simulink model "FSAC2021_V1"  (R2014a)
settings: Solver=FixedStepDiscrete  StartTime=0.0  StopTime=inf  FixedStep=0.0005  RelTol=1e-3
model workspace (MAT data in the model file):
  MCOS : class17 (value not decoded)
  MCOS : class17 (value not decoded)
  MCOS : class17 (value not decoded)
  MCOS : class17 (value not decoded)
  MCOS : class17 (value not decoded)
  MCOS : class17 (value not decoded)
  MCOS : class17 (value not decoded)
  MCOS : class17 (value not decoded)
  MCOS : class17 (value not decoded)
  MCOS : class17 (value not decoded)
  MCOS : class17 (value not decoded)
  MCOS : class17 (value not decoded)
  MCOS : class17 (value not decoded)
  MCOS : class17 (value not decoded)
  MCOS : class17 (value not decoded)
  MCOS : class17 (value not decoded)
  MCOS : class17 (value not decoded)
  MCOS : class17 (value not decoded)
  MCOS : class17 (value not decoded)
  BUZZER_START = 1
  MCOS : class17 (value not decoded)
  MCOS : class17 (value not decoded)
  MCOS : class17 (value not decoded)
  MCOS : class17 (value not decoded)
  MCOS : class17 (value not decoded)
  MCOS : class17 (value not decoded)
  MCOS : class17 (value not decoded)
  MCOS : class17 (value not decoded)
  MCOS : class17 (value not decoded)
  MCOS : class17 (value not decoded)
  MCOS : class17 (value not decoded)
  MCOS : class17 (value not decoded)
  MCOS : class17 (value not decoded)
  MCOS : class17 (value not decoded)
  MCOS : class17 (value not decoded)
  MCOS : class17 (value not decoded)
  MCOS : class17 (value not decoded)
  MCOS : class17 (value not decoded)
  MCOS : class17 (value not decoded)
  MCOS : class17 (value not decoded)
  MCOS : class17 (value not decoded)
  MCOS : class17 (value not decoded)
  MCOS : class17 (value not decoded)
  MCOS : class17 (value not decoded)
  MCOS : class17 (value not decoded)
  MCOS : class17 (value not decoded)
  MCOS : class17 (value not decoded)
  MCOS : class17 (value not decoded)
  MCOS : class17 (value not decoded)
  MCOS : class17 (value not decoded)
  MCOS : class17 (value not decoded)
  MCOS : class17 (value not decoded)
  MCOS : class17 (value not decoded)
  MCOS : class17 (value not decoded)
  MCOS : class17 (value not decoded)
  MCOS : class17 (value not decoded)
  MCOS : class17 (value not decoded)
  MCOS : class17 (value not decoded)
  Brake = 11
  MCOS : class17 (value not decoded)
  MCOS : class17 (value not decoded)
  MCOS : class17 (value not decoded)
  MCOS : class17 (value not decoded)
  MCOS : class17 (value not decoded)
  MCOS : class17 (value not decoded)
  MCOS : class17 (value not decoded)
  MCOS : class17 (value not decoded)
  Sensor_Acc_b = 101.85
  Sensor_Acc_k = -0.0185
  Str_Sen_Orig_Angle = -341
  MCOS : class17 (value not decoded)
  Tire_D = 0.47
  T = 0.05
libraries: simulink x189, ec55xxlib x135
(part 2 of 9)

== system FSAC2021_V1/CAN_SEND/Subsystem2 ==
  Brk_Mtr_GoalPos : Inport
  Acc_Cmd : Inport  Port=2
  function : TriggerPort  TriggerType=function-call
  BCU_MTR_MOVE_AB : Subsystem
  CANTransmit3 : ec55xxlib/RapidECU_U2/07CANCommucation/CANTransmit  canmodule=A  canbuffer=58  canmessageid=358  canmessagetype=Standard(11-bit ID)  datalength=4  sampletime=-1
  CANTransmit4 : ec55xxlib/RapidECU_U2/07CANCommucation/CANTransmit  canmodule=B  canbuffer=15  canmessageid=2197885092  canmessagetype=Extended(29-bit ID)  datalength=2  sampletime=-1
  Data Type Conversion17 : DataTypeConversion
  MOTOR_SPEED_CONTROL : Subsystem
  MeaModule : ec55xxlib/RapidECU_U2/11Calibration/MeaModule  signal=To_MOTOR_OK
  MeaModule1 : ec55xxlib/RapidECU_U2/11Calibration/MeaModule  signal=ACC
  MeaModule8 : ec55xxlib/RapidECU_U2/11Calibration/MeaModule  signal=pulses
  Terminator3 : Terminator
  Terminator4 : Terminator
  wires:
  Brk_Mtr_GoalPos/1 -> MeaModule8/1
  MOTOR_SPEED_CONTROL/1(output) -> CANTransmit4/1
  MeaModule1/1 -> MOTOR_SPEED_CONTROL/1(Drive_Speed_Control_in)
  MeaModule/1 -> Terminator4/1
  Acc_Cmd/1 -> MeaModule1/1
  CANTransmit3/1 -> Terminator3/1
  BCU_MTR_MOVE_AB/1(output) -> CANTransmit3/1
  CANTransmit4/1 -> MeaModule/1
  Data Type Conversion17/1 -> BCU_MTR_MOVE_AB/1(Brake_mtr_goalpos_in)
  MeaModule8/1 -> Data Type Conversion17/1

== system FSAC2021_V1/CAN_SEND/Subsystem3 ==
  BCU_STATUS_READ : Subsystem
  CANTransmit1 : ec55xxlib/RapidECU_U2/07CANCommucation/CANTransmit  canmodule=B  canbuffer=13  canmessageid=2181107875  canmessagetype=Extended(29-bit ID)  datalength=8  sampletime=0.05
  CANTransmit6 : ec55xxlib/RapidECU_U2/07CANCommucation/CANTransmit  canmodule=A  canbuffer=59  canmessageid=382  canmessagetype=Standard(11-bit ID)  datalength=2  sampletime=0.01
  Constant : Constant  Value=2
  Constant1 : Constant
  Data Type Conversion : DataTypeConversion
  MOTOR_READ_SPEED : Subsystem
  MeaModule1 : ec55xxlib/RapidECU_U2/11Calibration/MeaModule  signal=read_speed
  MeaModule2 : ec55xxlib/RapidECU_U2/11Calibration/MeaModule  signal=Read_BCU
  Terminator1 : Terminator
  Terminator6 : Terminator
  wires:
  CANTransmit6/1 -> MeaModule2/1
  Constant/1 -> BCU_STATUS_READ/1(status_reg_num_in)
  Constant1/1 -> BCU_STATUS_READ/2(status_reg_addr_start_in)
  BCU_STATUS_READ/1(output) -> CANTransmit6/1
  MeaModule2/1 -> Terminator6/1
  MOTOR_READ_SPEED/1(output) -> Data Type Conversion/1
  CANTransmit1/1 -> MeaModule1/1
  Data Type Conversion/1 -> CANTransmit1/1
  MeaModule1/1 -> Terminator1/1

== system FSAC2021_V1/Controller/200ms_Duty ==
  LED_Blue_Flag : Inport
  LED_Yellow_Flag : Inport  Port=2
  Buzzer_Flag : Inport  Port=3
  function : TriggerPort  TriggerType=function-call
  Light_Subsystem : Subsystem  TreatAsAtomicUnit=on
  Light_Subsystem1 : Subsystem  TreatAsAtomicUnit=on
  Light_Subsystem2 : Subsystem  TreatAsAtomicUnit=on
  MeaModule : ec55xxlib/RapidECU_U2/11Calibration/MeaModule  signal=blue
  Blue_Light_Pin : Outport
  Yellow_Light_Pin : Outport  Port=2
  Buzzer_Pin : Outport  Port=3
  Buzzer_Overflag : Outport  Port=4
  wires:
  LED_Yellow_Flag/1 -> Light_Subsystem1/1(Light_Status)
  Light_Subsystem1/1(Light_Output) -> Yellow_Light_Pin/1
  LED_Blue_Flag/1 -> Light_Subsystem/1(Light_Status)
  Light_Subsystem/1(Light_Output) -> MeaModule/1
  Buzzer_Flag/1 -> Light_Subsystem2/1(Buzzer_Flag)
  Light_Subsystem2/1(Buzzer_Pin) -> Buzzer_Pin/1
  Light_Subsystem2/2(Buzzer_Overflag) -> Buzzer_Overflag/1
  MeaModule/1 -> Blue_Light_Pin/1

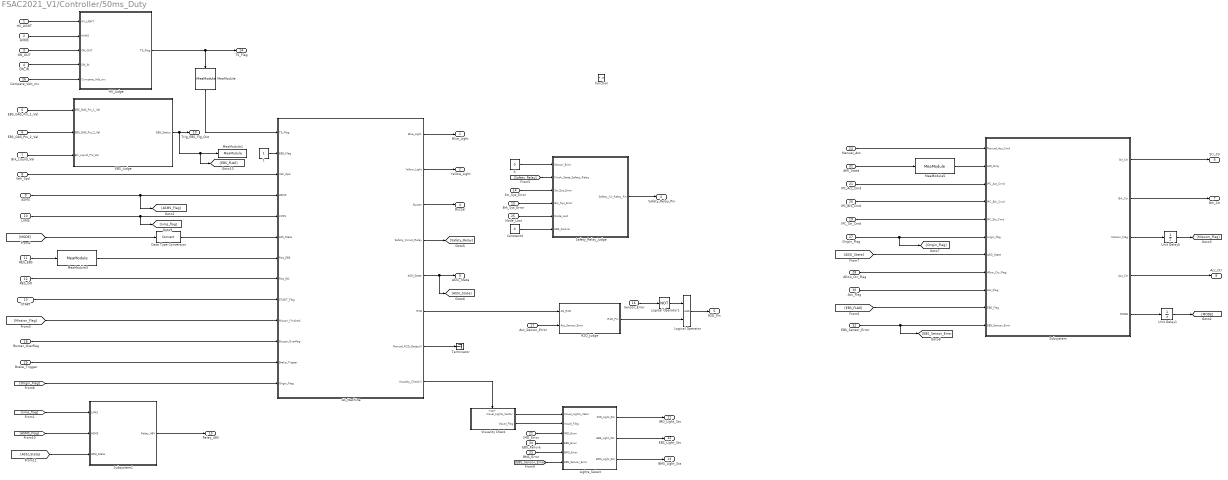
== system FSAC2021_V1/Controller/50ms_Duty ==
  HV_LIGHT : Inport
  HVMS : Inport  Port=2
  ON_OUT : Inport  Port=3
  ON_IN : Inport  Port=4
  EBS_GAS_Prs_1_Val : Inport  Port=5
  EBS_GAS_Prs_2_Val : Inport  Port=6
  Brk_Liquid_Val : Inport  Port=7
  Veh_Spd : Inport  Port=8
  ASMS : Inport  Port=9
  LVMS : Inport  Port=10
  RES_EBS : Inport  Port=11
  RES_GO : Inport  Port=12
  START : Inport  Port=13
  Str_Sys_Error : Inport  Port=14
  Brk_Sys_Error : Inport  Port=15
  Sensor_Error : Inport  Port=16
  Acc_Sensor_Error : Inport  Port=17
  Buzzer_Overflag : Inport  Port=18
  IPC_Str_Cmd : Inport  Port=19
  IPC_Brk_Cmd : Inport  Port=20
  IPC_Acc_Cmd : Inport  Port=21
  IMD_Error : Inport  Port=22
  BMS_Error : Inport  Port=23
  Manual_Acc : Inport  Port=24
  Node_Lost : Inport  Port=25
  Compare_Volt_mv : Inport  Port=26
  Origin_Flag : Inport  Port=27
  Allow_Ctr_Flag : Inport  Port=28
  "Brake_Trigger " : Inport  Port=29
  Acc_Flag : Inport  Port=30
  AMI_State : Inport  Port=31
  EBS_Sensor_Error : Inport  Port=32
  EBS_Failure : Inport  Port=33
  function : TriggerPort  TriggerType=function-call
  1 : Constant  OutDataTypeStr=uint8
  4 : Constant  Value=0  OutDataTypeStr=uint8
  AS_Machine : Stateflow chart  TreatAsAtomicUnit=on
  Constant2 : Constant  Value=0
  Data Type Conversion : DataTypeConversion
  EBS_Judge : Subsystem
  "HV_Judge " : Subsystem
  Lights_Select : Subsystem
  Logical Operator : Logic  AllPortsSameDT=off  OutDataTypeStr=boolean
  Logical Operator1 : Logic  Operator=NOT  AllPortsSameDT=off  OutDataTypeStr=boolean
  MeaModule : ec55xxlib/RapidECU_U2/11Calibration/MeaModule  signal=TS_Flag
  MeaModule1 : ec55xxlib/RapidECU_U2/11Calibration/MeaModule  signal=EBS_Status
  MeaModule3 : ec55xxlib/RapidECU_U2/11Calibration/MeaModule  signal=RES_EBS
  MeaModule5 : ec55xxlib/RapidECU_U2/11Calibration/MeaModule  signal=AMI_State
  R2D_Judge : Subsystem
  Safety_Relay_Judge : Subsystem
  Subsystem : Subsystem
  Subsystem1 : Subsystem
  Terminator : Terminator
  Unit Delay1 : UnitDelay  SampleTime=-1
  Unit Delay5 : UnitDelay  SampleTime=-1
  Visuality Check : Subsystem  TreatAsAtomicUnit=on
  Blue_Light : Outport
  Yellow_Light : Outport  Port=2
  Buzzer : Outport  Port=3
  Safety_Relay_Pin : Outport  Port=4
  R2D_Pin : Outport  Port=5
  Str_Ctr : Outport  Port=6
  Brk_Ctr : Outport  Port=7
  Acc_Ctr : Outport  Port=8
  ASSI_State : Outport  Port=9
  Trig_EBS_Flg_Out : Outport  Port=10
  IMD_Light_Sts : Outport  Port=11
  EBS_Light_Sts : Outport  Port=12
  BMS_Light_Sts : Outport  Port=13
  TS_Flag : Outport  Port=14
  Relay_48V : Outport  Port=15
  wires:
  HV_LIGHT/1 -> "HV_Judge "/1(HV_LIGHT)
  HVMS/1 -> "HV_Judge "/2(HVMS)
  EBS_GAS_Prs_2_Val/1 -> EBS_Judge/2(EBS_GAS_Prs_2_Val)
  EBS_GAS_Prs_1_Val/1 -> EBS_Judge/1(EBS_GAS_Prs_1_Val)
  EBS_Judge/1(EBS_Status) -> Trig_EBS_Flg_Out/1, [EBS_FLAG], MeaModule1/1
  ASMS/1 -> [ASMS_Flag], AS_Machine/4(ASMS)
  LVMS/1 -> [lvms_flag], AS_Machine/5(LVMS)
  ON_OUT/1 -> "HV_Judge "/3(ON_OUT)
  AS_Machine/2(Yellow_Light) -> Yellow_Light/1
  AS_Machine/1(Blue_Light) -> Blue_Light/1
  AS_Machine/3(Buzzer) -> Buzzer/1
  AS_Machine/6(R2D) -> R2D_Judge/1(AS_R2D)
  Buzzer_Overflag/1 -> AS_Machine/11(Buzzer_Overflag)
  ON_IN/1 -> "HV_Judge "/4(ON_IN)
  RES_EBS/1 -> MeaModule3/1
  Safety_Relay_Judge/1(Safety_Cir_Relay_Pin) -> Safety_Relay_Pin/1
  Acc_Sensor_Error/1 -> R2D_Judge/2(Acc_Sensor_Error)
  IPC_Str_Cmd/1 -> Subsystem/5(IPC_Str_Cmd)
  IPC_Brk_Cmd/1 -> Subsystem/4(IPC_Brk_Cmd)
  IPC_Acc_Cmd/1 -> Subsystem/3(IPC_Acc_Cmd)
  Subsystem/1(Str_Ctr) -> Str_Ctr/1
  Subsystem/2(Brk_Ctr) -> Brk_Ctr/1
  Brk_Liquid_Val/1 -> EBS_Judge/3(Brk_Liquid_Prs_Val)
  Visuality Check/1(Visual_Lights_Vector) -> Lights_Select/1(Visual_Lights_Vetor)
  Visuality Check/2(Visual_Flag) -> Lights_Select/2(Visual_Flag)
  IMD_Error/1 -> Lights_Select/3(IMD_Error)
  EBS_Failure/1 -> Lights_Select/4(EBS_Error)
  BMS_Error/1 -> Lights_Select/5(BMS_Error)
  Lights_Select/2(EBS_Light_Sts) -> EBS_Light_Sts/1
  Lights_Select/1(IMD_Light_Sts) -> IMD_Light_Sts/1
  Lights_Select/3(BMS_Light_Sts) -> BMS_Light_Sts/1
  AS_Machine/8(Visuality_Check()) -> Visuality Check/Trigger
  Manual_Acc/1 -> Subsystem/1(Manual_Acc_Cmd)
  AS_Machine/5(ASSI_State) -> [ASSI_State], ASSI_State/1
  Str_Sys_Error/1 -> Safety_Relay_Judge/3(Str_Sys_Error)
  Brk_Sys_Error/1 -> Safety_Relay_Judge/4(Brk_Sys_Error)
  Veh_Spd/1 -> AS_Machine/3(Veh_Spd)
  MeaModule/1 -> AS_Machine/1(TS_Flag)
  Compare_Volt_mv/1 -> "HV_Judge "/5(Compare_Volt_mv)
  "HV_Judge "/1(TS_Flag) -> MeaModule/1, TS_Flag/1
  START/1 -> AS_Machine/9(START_Flag)
  Origin_Flag/1 -> [Origin_Flag], Subsystem/6(origin_flag)
  Unit Delay5/1 -> [Mission_Flag]
  Subsystem/4(Acc_Ctr) -> Acc_Ctr/1
  RES_GO/1 -> AS_Machine/8(Res_GO)
  MeaModule3/1 -> AS_Machine/7(Res_EBS)
  [Mission_Flag] -> AS_Machine/10(Misson_Finished)
  Subsystem/3(Mission_Flag) -> Unit Delay5/1
  "Brake_Trigger "/1 -> AS_Machine/12(Brake_Trigeer)
  Constant2/1 -> Safety_Relay_Judge/6(EBS_Failure)
  Acc_Flag/1 -> Subsystem/9(Acc_Flag)
  R2D_Judge/1(R2D_Pin) -> Logical Operator/2
  Logical Operator/1 -> R2D_Pin/1
  Sensor_Error/1 -> Logical Operator1/1
  Logical Operator1/1 -> Logical Operator/1
  Allow_Ctr_Flag/1 -> Subsystem/8(Allow_Ctr_Flag)
  4/1 -> Safety_Relay_Judge/1(Sensor_Error)
  AS_Machine/4(Safety_Circuit_Relay) -> [Safety_Relay]
  [Safety_Relay] -> Safety_Relay_Judge/2(Finish_State_Safety_Relay)
  [ASSI_State] -> Subsystem/7(ASSI_State)
  AMI_State/1 -> MeaModule5/1
  MeaModule5/1 -> Subsystem/2(AMI_Duty)
  Subsystem/5(MODE) -> Unit Delay1/1
  Unit Delay1/1 -> [MODE]
  [MODE] -> Data Type Conversion/1
  Data Type Conversion/1 -> AS_Machine/6(AMI_State)
  [Origin_Flag] -> AS_Machine/13(Origin_Flag)
  EBS_Sensor_Error/1 -> [EBS_Sensor_Error], Subsystem/11(EBS_Sensor_Error)
  [EBS_Sensor_Error] -> Lights_Select/6(EBS_Sensor_Error)
  Node_Lost/1 -> Safety_Relay_Judge/5(Node_Lost)
  [lvms_flag] -> Subsystem1/1(LVMS)
  [ASMS_Flag] -> Subsystem1/2(ASMS)
  [ASSI_State] -> Subsystem1/3(ASSI_State)
  Subsystem1/1(Relay_48V) -> Relay_48V/1
  [EBS_FLAG] -> Subsystem/10(EBS_Flag)
  AS_Machine/7(Manual_R2D_Detect()) -> Terminator/1
  1/1 -> AS_Machine/2(EBS_Flag)

== system FSAC2021_V1/Controller/BCU_Controller ==
  note: 任何控制源禁止在Allow_Ctrl_Flg未置1的时候控制车辆
  Brk_Cmd : Inport
  Brk_Mtr_Enable_Flg : Inport  Port=2
  ASSI_State : Inport  Port=3
  function : TriggerPort  TriggerType=function-call
  BCU_Strategy : Stateflow chart
  Brk_Move : Subsystem
  Constant1 : Constant
  MeaModule : ec55xxlib/RapidECU_U2/11Calibration/MeaModule  signal=Brk_Enable_Flag
  Allow_Ctrl_Flg : Outport
  Brk_Mtr_Origin_funCall : Outport  Port=2
  Brk_Mtr_Enable_funCall : Outport  Port=3
  Brk_Mtr_GoalPos : Outport  Port=4
  wires:
  Brk_Mtr_Enable_Flg/1 -> MeaModule/1
  Constant1/1 -> BCU_Strategy/3(Brk_Mtr_Origin_Flag)
  BCU_Strategy/2(Brk_Ctrl_State) -> Brk_Move/1(Brk_Ctrl_State)
  ASSI_State/1 -> BCU_Strategy/2(ASSI_State)
  BCU_Strategy/1(Allow_Ctrl_Flg) -> Allow_Ctrl_Flg/1
  BCU_Strategy/3(Brk_Mtr_BackOrigin()) -> Brk_Mtr_Origin_funCall/1
  BCU_Strategy/4(Brk_Mtr_Enable()) -> Brk_Mtr_Enable_funCall/1
  Brk_Move/1(Brk_Mtr_GoalPos) -> Brk_Mtr_GoalPos/1
  Brk_Cmd/1 -> Brk_Move/2(Brk_Cmd)
  MeaModule/1 -> BCU_Strategy/1(Brk_Mtr_Enable_Flg)

== system FSAC2021_V1/Controller/SteerCtr ==
  Str_Snr_Ang : Inport
  Steer_Cmd : Inport  Port=2
  Str_Status : Inport  Port=3
  ASSI_State : Inport  Port=4
  function : TriggerPort  TriggerType=function-call
  Chart : Stateflow chart  SystemSampleTime=0.01
  Data Type Conversion{,1..3} (4 alike) : DataTypeConversion
  MeaModule : ec55xxlib/RapidECU_U2/11Calibration/MeaModule  signal=Back_Angle
  MeaModule1 : ec55xxlib/RapidECU_U2/11Calibration/MeaModule  signal=enflag
  MeaModule2 : ec55xxlib/RapidECU_U2/11Calibration/MeaModule  signal=flag
  MeaModule3 : ec55xxlib/RapidECU_U2/11Calibration/MeaModule  signal=Str
  Subsystem3 : Subsystem
  Terminator : Terminator
  Terminator1 : Terminator
  NMT_nodeorder : Outport
  NMT_nodectrl : Outport  Port=2
  Enable_Operation_Ctrl : Outport  Port=3
  Quick_Stop_Ctrl : Outport  Port=4
  Enable_Voltage_Ctrl : Outport  Port=5
  Halt_Ctrl : Outport  Port=6
  Switch_On_Ctrl : Outport  Port=7
  Abs_or_Rel_Ctrl : Outport  Port=8
  New_Set_Point_Ctrl : Outport  Port=9
  Position_set : Outport  Port=10
  Encoder_Msg_Data : Outport  Port=11
  TmtNNMTCAN : Outport  Port=12
  TmtRPDO1CAN : Outport  Port=13
  TmtSDOCAN : Outport  Port=14
  Original_Flag : Outport  Port=15
  Fault_Reset : Outport  Port=16
  wires:
  Str_Status/1 -> Data Type Conversion1/1
  Data Type Conversion3/1 -> Subsystem3/1(In1)
  ASSI_State/1 -> Data Type Conversion/1
  Data Type Conversion2/1 -> MeaModule3/1
  Data Type Conversion/1 -> Chart/3(ASSI_State)
  Data Type Conversion1/1 -> Chart/4(Str_Status)
  Chart/1(NMT_nodeorder) -> NMT_nodeorder/1
  Chart/2(NMT_nodectrl) -> NMT_nodectrl/1
  Chart/3(Enable_Operation_Ctrl) -> Enable_Operation_Ctrl/1
  Chart/4(Quick_Stop_Ctrl) -> Quick_Stop_Ctrl/1
  Chart/5(Enable_Voltage_Ctrl) -> Enable_Voltage_Ctrl/1
  Chart/6(Halt_Ctrl) -> Halt_Ctrl/1
  Chart/7(Switch_On_Ctrl) -> Switch_On_Ctrl/1
  Chart/8(Abs_or_Rel_Ctrl) -> Abs_or_Rel_Ctrl/1
  Chart/9(New_Set_Point_Ctrl) -> New_Set_Point_Ctrl/1
  Chart/11(Encoder_Msg_Data) -> Encoder_Msg_Data/1
  Chart/12(Original_Flag) -> Original_Flag/1
  Chart/16(TmtNMTCAN()) -> TmtNNMTCAN/1
  Chart/17(TmtRPDO1CAN()) -> TmtRPDO1CAN/1
  Chart/18(TmtSDOCAN()) -> TmtSDOCAN/1
  Subsystem3/1(Out1) -> MeaModule/1
  MeaModule/1 -> Chart/1(Origin_Back_Angle)
  Str_Snr_Ang/1 -> Data Type Conversion3/1
  Chart/13(Fault_Resrt) -> Fault_Reset/1
  Chart/10(Position_set) -> Position_set/1
  Chart/14(flag) -> MeaModule2/1
  MeaModule2/1 -> Terminator/1
  MeaModule3/1 -> Chart/2(Steer_Go_Angle)
  Chart/15(enflag) -> MeaModule1/1
  MeaModule1/1 -> Terminator1/1
  Steer_Cmd/1 -> Data Type Conversion2/1

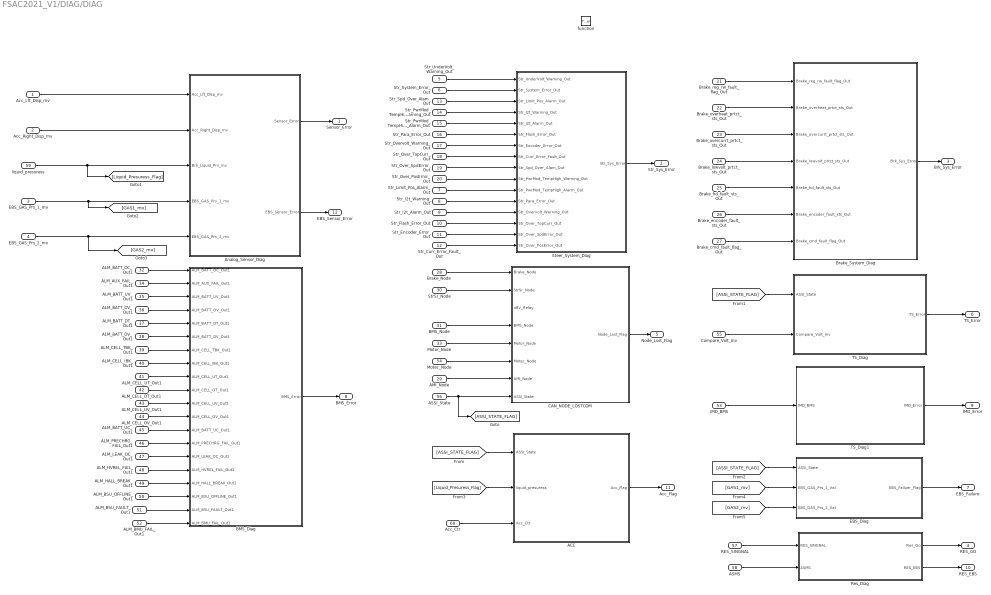
== system FSAC2021_V1/DIAG/DIAG ==
  Acc_Lft_Disp_mv : Inport
  Acc_Right_Disp_mv : Inport  Port=2
  EBS_GAS_Prs_1_mv : Inport  Port=3
  EBS_GAS_Prs_2_mv : Inport  Port=4
  Str_UnderVolt_Warning_Out : Inport  Port=5
  Str_System_Error_Out : Inport  Port=6
  Str_Limit_Pos_Alarm_Out : Inport  Port=7
  Str_I2t_Warning_Out : Inport  Port=8
  Str_I2t_Alarm_Out : Inport  Port=9
  Str_Flash_Error_Out : Inport  Port=10
  Str_Encoder_Error_Out : Inport  Port=11
  Str_Curr_Error_Fault_Out : Inport  Port=12
  Str_Spd_Over_Alam_Out : Inport  Port=13
  Str_PwrMod_TempHigh_Warning_Out : Inport  Port=14
  Str_PwrMod_TempHigh_Alarm_Out : Inport  Port=15
  Str_Para_Error_Out : Inport  Port=16
  Str_Overvolt_Warning_Out : Inport  Port=17
  Str_Over_TopCurr_Out : Inport  Port=18
  Str_Over_SpdError_Out : Inport  Port=19
  Str_Over_PosError_Out : Inport  Port=20
  Brake_reg_rw_fault_flag_Out : Inport  Port=21
  Brake_overheat_prtct_sts_Out : Inport  Port=22
  Brake_overcurrt_prtct_sts_Out : Inport  Port=23
  Brake_lowvolt_prtct_sts_Out : Inport  Port=24
  Brake_hd_fault_sts_Out : Inport  Port=25
  Brake_encoder_fault_sts_Out : Inport  Port=26
  Brake_cmd_fault_flag_Out : Inport  Port=27
  Brake_Node : Inport  Port=28
  AMI_Node : Inport  Port=29
  StrSr_Node : Inport  Port=30
  BMS_Node : Inport  Port=31
  ALM_BATT_OC_Out1 : Inport  Port=32
  Motor_Node : Inport  Port=33
  ALM_AUX_FAIL_Out1 : Inport  Port=34
  ALM_BATT_UV_Out1 : Inport  Port=35
  ALM_BATT_OV_Out1 : Inport  Port=36
  ALM_BATT_DT_Out1 : Inport  Port=37
  ALM_BATT_DV_Out1 : Inport  Port=38
  ALM_CELL_TBK_Out1 : Inport  Port=39
  ALM_CELL_IBK_Out1 : Inport  Port=40
  ALM_CELL_UT_Out1 : Inport  Port=41
  ALM_CELL_OT_Out1 : Inport  Port=42
  ALM_CELL_UV_Out1 : Inport  Port=43
  ALM_CELL_OV_Out1 : Inport  Port=44
  ALM_BATT_UC_Out1 : Inport  Port=45
  ALM_PRECHRG_FAIL_Out1 : Inport  Port=46
  ALM_LEAK_OC_Out1 : Inport  Port=47
  ALM_HVREL_FAIL_Out1 : Inport  Port=48
  ALM_HALL_BREAK_Out1 : Inport  Port=49
  ALM_BSU_OFFLINE_Out1 : Inport  Port=50
  ALM_BSU_FAULT_Out1 : Inport  Port=51
  ALM_BMU_FAIL_Out1 : Inport  Port=52
  "IMD_BMS " : Inport  Port=53
  Motec_Node : Inport  Port=54
  Compare_Volt_mv : Inport  Port=55
  ASSI_State : Inport  Port=56
  RES_SINGNAL : Inport  Port=57
  ASMS : Inport  Port=58
  liquid_presuress : Inport  Port=59
  Acc_Ctr : Inport  Port=60
  function : TriggerPort  TriggerType=function-call
  ACC : Subsystem
  Analog_Sensor_Diag : Subsystem
  BMS_Diag : Subsystem
  Brake_System_Diag : Subsystem
  CAN_NODE_LOSTCOM : Subsystem
  EBS_Diag : Subsystem
  Res_Diag : Subsystem
  Steer_System_Diag : Subsystem
  TS_Diag : Subsystem
  TS_Diag1 : Subsystem
  Sensor_Error : Outport
  Str_Sys_Error : Outport  Port=2
  Brk_Sys_Error : Outport  Port=3
  RES_GO : Outport  Port=4
  Node_Lost_Flag : Outport  Port=5
  TS_Error : Outport  Port=6
  EBS_Failure : Outport  Port=7
  "BMS_Error " : Outport  Port=8
  IMD_Error : Outport  Port=9
  RES_EBS : Outport  Port=10
  Acc_Flag : Outport  Port=11
  EBS_Sensor_Error : Outport  Port=12
  wires:
  Str_UnderVolt_Warning_Out/1 -> Steer_System_Diag/1(Str_UnderVolt_Warning_Out)
  Str_System_Error_Out/1 -> Steer_System_Diag/2(Str_System_Error_Out)
  Str_Spd_Over_Alam_Out/1 -> Steer_System_Diag/3(Str_Limit_Pos_Alarm_Out)
  Str_PwrMod_TempHigh_Warning_Out/1 -> Steer_System_Diag/4(Str_I2t_Warning_Out)
  Str_PwrMod_TempHigh_Alarm_Out/1 -> Steer_System_Diag/5(Str_I2t_Alarm_Out)
  Str_Overvolt_Warning_Out/1 -> Steer_System_Diag/7(Str_Encoder_Error_Out)
  Str_Over_TopCurr_Out/1 -> Steer_System_Diag/8(Str_Curr_Error_Fault_Out)
  Str_Para_Error_Out/1 -> Steer_System_Diag/6(Str_Flash_Error_Out)
  Str_Over_SpdError_Out/1 -> Steer_System_Diag/9(Str_Spd_Over_Alam_Out)
  Str_Over_PosError_Out/1 -> Steer_System_Diag/10(Str_PwrMod_TempHigh_Warning_Out)
  Str_Limit_Pos_Alarm_Out/1 -> Steer_System_Diag/11(Str_PwrMod_TempHigh_Alarm_Out)
  Str_I2t_Warning_Out/1 -> Steer_System_Diag/12(Str_Para_Error_Out)
  Str_I2t_Alarm_Out/1 -> Steer_System_Diag/13(Str_Overvolt_Warning_Out)
  Str_Flash_Error_Out/1 -> Steer_System_Diag/14(Str_Over_TopCurr_Out)
  Str_Encoder_Error_Out/1 -> Steer_System_Diag/15(Str_Over_SpdError_Out)
  Str_Curr_Error_Fault_Out/1 -> Steer_System_Diag/16(Str_Over_PosError_Out)
  Steer_System_Diag/1(Str_Sys_Error) -> Str_Sys_Error/1
  Brake_overcurrt_prtct_sts_Out/1 -> Brake_System_Diag/3(Brake_overcurrt_prtct_sts_Out)
  Brake_overheat_prtct_sts_Out/1 -> Brake_System_Diag/2(Brake_overheat_prtct_sts_Out)
  Brake_lowvolt_prtct_sts_Out/1 -> Brake_System_Diag/4(Brake_lowvolt_prtct_sts_Out)
  Brake_reg_rw_fault_flag_Out/1 -> Brake_System_Diag/1(Brake_reg_rw_fault_flag_Out)
  Brake_hd_fault_sts_Out/1 -> Brake_System_Diag/5(Brake_hd_fault_sts_Out)
  Brake_encoder_fault_sts_Out/1 -> Brake_System_Diag/6(Brake_encoder_fault_sts_Out)
  Brake_cmd_fault_flag_Out/1 -> Brake_System_Diag/7(Brake_cmd_fault_flag_Out)
  Brake_System_Diag/1(Brk_Sys_Error) -> Brk_Sys_Error/1
  Acc_Right_Disp_mv/1 -> Analog_Sensor_Diag/2(Acc_Right_Disp_mv)
  Acc_Lft_Disp_mv/1 -> Analog_Sensor_Diag/1(Acc_Lft_Disp_mv)
  Analog_Sensor_Diag/1(Sensor_Error) -> Sensor_Error/1
  CAN_NODE_LOSTCOM/1(Node_Lost_Flag) -> Node_Lost_Flag/1
  TS_Diag/1(TS_Error) -> TS_Error/1
  EBS_GAS_Prs_1_mv/1 -> Analog_Sensor_Diag/4(EBS_GAS_Prs_1_mv), [GAS1_mv]
  EBS_GAS_Prs_2_mv/1 -> [GAS2_mv], Analog_Sensor_Diag/5(EBS_GAS_Prs_2_mv)
  EBS_Diag/1(EBS_Failuer_Flag) -> EBS_Failure/1
  ASSI_State/1 -> [ASSI_STATE_FLAG], CAN_NODE_LOSTCOM/8(ASSI_State)
  ALM_BATT_OC_Out1/1 -> BMS_Diag/1(ALM_BATT_OC_Out1)
  ALM_AUX_FAIL_Out1/1 -> BMS_Diag/2(ALM_AUX_FAIL_Out1)
  ALM_BATT_UV_Out1/1 -> BMS_Diag/3(ALM_BATT_UV_Out1)
  ALM_BATT_OV_Out1/1 -> BMS_Diag/4(ALM_BATT_OV_Out1)
  ALM_BATT_DT_Out1/1 -> BMS_Diag/5(ALM_BATT_DT_Out1)
  ALM_BATT_DV_Out1/1 -> BMS_Diag/6(ALM_BATT_DV_Out1)
  ALM_CELL_TBK_Out1/1 -> BMS_Diag/7(ALM_CELL_TBK_Out1)
  ALM_CELL_IBK_Out1/1 -> BMS_Diag/8(ALM_CELL_IBK_Out1)
  ALM_CELL_UT_Out1/1 -> BMS_Diag/9(ALM_CELL_UT_Out1)
  ALM_CELL_OT_Out1/1 -> BMS_Diag/10(ALM_CELL_OT_Out1)
  ALM_CELL_UV_Out1/1 -> BMS_Diag/11(ALM_CELL_UV_Out1)
  ALM_CELL_OV_Out1/1 -> BMS_Diag/12(ALM_CELL_OV_Out1)
  ALM_BATT_UC_Out1/1 -> BMS_Diag/13(ALM_BATT_UC_Out1)
  ALM_PRECHRG_FAIL_Out1/1 -> BMS_Diag/14(ALM_PRECHRG_FAIL_Out1)
  ALM_LEAK_OC_Out1/1 -> BMS_Diag/15(ALM_LEAK_OC_Out1)
  ALM_HVREL_FAIL_Out1/1 -> BMS_Diag/16(ALM_HVREL_FAIL_Out1)
  ALM_HALL_BREAK_Out1/1 -> BMS_Diag/17(ALM_HALL_BREAK_Out1)
  ALM_BSU_OFFLINE_Out1/1 -> BMS_Diag/18(ALM_BSU_OFFLINE_Out1)
  ALM_BSU_FAULT_Out1/1 -> BMS_Diag/19(ALM_BSU_FAULT_Out1)
  ALM_BMU_FAIL_Out1/1 -> BMS_Diag/20(ALM_BMU_FAIL_Out1)
  BMS_Diag/1("BMS_Error ") -> "BMS_Error "/1
  "IMD_BMS "/1 -> TS_Diag1/1("IMD_BMS ")
  TS_Diag1/1(IMD_Error) -> IMD_Error/1
  Brake_Node/1 -> CAN_NODE_LOSTCOM/1(Brake_Node)
  Motor_Node/1 -> CAN_NODE_LOSTCOM/5(Motor_Node)
  StrSr_Node/1 -> CAN_NODE_LOSTCOM/2(StrSr_Node)
  BMS_Node/1 -> CAN_NODE_LOSTCOM/4(BMS_Node)
  Motec_Node/1 -> CAN_NODE_LOSTCOM/6(Motec_Node)
  Compare_Volt_mv/1 -> TS_Diag/2(Compare_Volt_mv)
  AMI_Node/1 -> CAN_NODE_LOSTCOM/7(AMI_Node)
  Res_Diag/1(Res_Go) -> RES_GO/1
  RES_SINGNAL/1 -> Res_Diag/1(RES_SINGNAL)
  ASMS/1 -> Res_Diag/2(ASMS)
  Res_Diag/2(RES_EBS) -> RES_EBS/1
  Acc_Ctr/1 -> ACC/3(Acc_Ctr)
  ACC/1(Acc_Flag) -> Acc_Flag/1
  liquid_presuress/1 -> Analog_Sensor_Diag/3(Brk_Liquid_Prs_mv), [Liquid_Presuress_Flag]
  Analog_Sensor_Diag/2(EBS_Sensor_Error) -> EBS_Sensor_Error/1
  [ASSI_STATE_FLAG] -> ACC/1(ASSI_State)
  [ASSI_STATE_FLAG] -> TS_Diag/1(ASSI_State)
  [ASSI_STATE_FLAG] -> EBS_Diag/1(ASSI_State)
  [Liquid_Presuress_Flag] -> ACC/2(liquid_presuress)
  [GAS1_mv] -> EBS_Diag/2(EBS_GAS_Prs_1_Val)
  [GAS2_mv] -> EBS_Diag/3(EBS_GAS_Prs_2_Val)

== system FSAC2021_V1/I//O_OutPut/Subsystem ==
  Blue_Light_Pin : Inport
  Yellow_Light_Pin : Inport  Port=2
  Buzzer_pin : Inport  Port=3
  Safety_Relay_Pin : Inport  Port=4
  Relay_48V_Pin : Inport  Port=5
  R2D_pin : Inport  Port=6
  IMD_Light : Inport  Port=7
  EBS_Light : Inport  Port=8
  BMS_Light : Inport  Port=9
  Liquid_Pressure : Inport  Port=10
  function : TriggerPort  TriggerType=function-call
  48V_Relay : ec55xxlib/RapidECU_U2/04PowerDriverSwitch/PowerDriverSwitch  channel=59: O_PWM2_LS1A8  sampletime=-1
  Blue_Pin : ec55xxlib/RapidECU_U2/04PowerDriverSwitch/PowerDriverSwitch  channel=114: O_PWM9_HS2A9  sampletime=-1
  Buzzer_Pin : ec55xxlib/RapidECU_U2/04PowerDriverSwitch/PowerDriverSwitch  channel=117: O_PWM11_HS2A9  sampletime=-1
  Compare To Constant : simulink/Logic and Bit Operations/Compare To Constant  relop=>=  const=30  OutDataTypeStr=boolean
  Constant : Constant
  Constant1 : Constant  Value=0
  Data Type Conversion{,1..4,6..10} (10 alike) : DataTypeConversion  OutDataTypeStr=boolean
  MeaModule : ec55xxlib/RapidECU_U2/11Calibration/MeaModule  signal=Stafe_Relay_pin
  MeaModule1 : ec55xxlib/RapidECU_U2/11Calibration/MeaModule  signal=R2D_Voltage
  MeaModule2 : ec55xxlib/RapidECU_U2/11Calibration/MeaModule  signal=Buzzer_pin
  MeaModule3 : ec55xxlib/RapidECU_U2/11Calibration/MeaModule  signal=V48_relay
  MeaModule4 : ec55xxlib/RapidECU_U2/11Calibration/MeaModule  signal=IMD
  MeaModule5 : ec55xxlib/RapidECU_U2/11Calibration/MeaModule  signal=EBS
  MeaModule6 : ec55xxlib/RapidECU_U2/11Calibration/MeaModule  signal=BMS_LIGHT
  MeaModule7 : ec55xxlib/RapidECU_U2/11Calibration/MeaModule  signal=light_blue
  MeaModule8 : ec55xxlib/RapidECU_U2/11Calibration/MeaModule  signal=brake_light
  R2D_Pin : ec55xxlib/RapidECU_U2/04PowerDriverSwitch/PowerDriverSwitch  channel=61: O_PWM4_LS1A8  sampletime=-1
  "Safety_Relay " : ec55xxlib/RapidECU_U2/04PowerDriverSwitch/PowerDriverSwitch  channel=58: O_PWM1_LS1A8  sampletime=-1
  Switch : Switch  Criteria=u2 > Threshold
  VCU_Valve1 : ec55xxlib/RapidECU_U2/04PowerDriverSwitch/PowerDriverSwitch  channel=82: O_PWM5_LS1A8  sampletime=-1
  VCU_Valve2 : ec55xxlib/RapidECU_U2/04PowerDriverSwitch/PowerDriverSwitch  channel=90: O_PWM6_LS1A8  sampletime=-1
  VCU_Valve3 : ec55xxlib/RapidECU_U2/04PowerDriverSwitch/PowerDriverSwitch  channel=92: O_PWM7_LS1A8  sampletime=-1
  VCU_Valve4 : ec55xxlib/RapidECU_U2/04PowerDriverSwitch/PowerDriverSwitch  channel=118: O_PWM12_HS2A9  sampletime=-1
  Yellow_Pin : ec55xxlib/RapidECU_U2/04PowerDriverSwitch/PowerDriverSwitch  channel=115: O_PWM10_HS2A9  sampletime=-1
  wires:
  Data Type Conversion1/1 -> Yellow_Pin/1
  Blue_Light_Pin/1 -> Data Type Conversion/1
  Buzzer_pin/1 -> Data Type Conversion2/1
  Data Type Conversion2/1 -> MeaModule2/1
  Data Type Conversion3/1 -> MeaModule/1
  Data Type Conversion4/1 -> MeaModule3/1
  Yellow_Light_Pin/1 -> Data Type Conversion1/1
  R2D_pin/1 -> Data Type Conversion6/1
  Data Type Conversion/1 -> MeaModule7/1
  Data Type Conversion9/1 -> MeaModule5/1
  MeaModule2/1 -> Buzzer_Pin/1
  EBS_Light/1 -> Data Type Conversion9/1
  BMS_Light/1 -> Data Type Conversion10/1
  Safety_Relay_Pin/1 -> Data Type Conversion3/1
  MeaModule/1 -> "Safety_Relay "/1
  Data Type Conversion8/1 -> MeaModule4/1
  MeaModule4/1 -> VCU_Valve1/1
  MeaModule3/1 -> 48V_Relay/1
  MeaModule5/1 -> VCU_Valve2/1
  MeaModule6/1 -> VCU_Valve3/1
  IMD_Light/1 -> Data Type Conversion8/1
  Data Type Conversion6/1 -> MeaModule1/1
  Data Type Conversion10/1 -> MeaModule6/1
  MeaModule1/1 -> R2D_Pin/1
  Relay_48V_Pin/1 -> Data Type Conversion4/1
  MeaModule7/1 -> Blue_Pin/1
  Data Type Conversion7/1 -> MeaModule8/1
  Switch/1 -> Data Type Conversion7/1
  Liquid_Pressure/1 -> Compare To Constant/1
  Compare To Constant/1 -> Switch/2
  Constant/1 -> Switch/1
  Constant1/1 -> Switch/3
  MeaModule8/1 -> VCU_Valve4/1

== system FSAC2021_V1/Input_Process/KL_Sig_Process ==
  FL_WhlSpd_Hz : Inport
  FR_WhlSpd_Hz : Inport  Port=2
  RL_WhlSpd_Hz : Inport  Port=3
  RR_WhlSpd_Hz : Inport  Port=4
  Acc_Lft_Disp_mv : Inport  Port=5
  Acc_Right_Disp_mv : Inport  Port=6
  Brk_Liquid_Prs_mv : Inport  Port=7
  EBS_GAS_Prs_1_mv : Inport  Port=8
  EBS_GAS_Prs_2_mv : Inport  Port=9
  function : TriggerPort  TriggerType=function-call
  Analog_Signal_Process : Subsystem
  Whl_Spd_Process : Subsystem
  Vel_Spd : Outport
  Whl_Spd_FL_Val : Outport  Port=2
  Whl_Spd_FF_Val : Outport  Port=3
  Whl_Spd_RL_Val : Outport  Port=4
  Whl_Spd_RR_Val : Outport  Port=5
  Acc_Lft_Disp_Val : Outport  Port=6
  Acc_Right_Disp_Val : Outport  Port=7
  Brk_Liquid_Prs_Val : Outport  Port=8
  EBS_GAS_Prs_1_Val : Outport  Port=9
  EBS_GAS_Prs_2_Val : Outport  Port=10
  ACC : Outport  Port=11
  wires:
  Whl_Spd_Process/2(Whl_Spd_FL_Val) -> Whl_Spd_FL_Val/1
  Whl_Spd_Process/3(Whl_Spd_FF_Val) -> Whl_Spd_FF_Val/1
  Whl_Spd_Process/4(Whl_Spd_RL_Val) -> Whl_Spd_RL_Val/1
  Whl_Spd_Process/5(Whl_Spd_RR_Val) -> Whl_Spd_RR_Val/1
  Whl_Spd_Process/1(Vel_Spd) -> Vel_Spd/1
  RR_WhlSpd_Hz/1 -> Whl_Spd_Process/4(RR_WhlSpd_Hz)
  RL_WhlSpd_Hz/1 -> Whl_Spd_Process/3(RL_WhlSpd_Hz)
  FR_WhlSpd_Hz/1 -> Whl_Spd_Process/2(FR_WhlSpd_Hz)
  FL_WhlSpd_Hz/1 -> Whl_Spd_Process/1(FL_WhlSpd_Hz)
  Analog_Signal_Process/3(Brk_Liquid_Prs_Val) -> Brk_Liquid_Prs_Val/1
  Analog_Signal_Process/4(EBS_GAS_Prs_1_Val) -> EBS_GAS_Prs_1_Val/1
  Analog_Signal_Process/5(EBS_GAS_Prs_2_Val) -> EBS_GAS_Prs_2_Val/1
  EBS_GAS_Prs_2_mv/1 -> Analog_Signal_Process/5(EBS_GAS_Prs_2_mv)
  EBS_GAS_Prs_1_mv/1 -> Analog_Signal_Process/4(EBS_GAS_Prs_1_mv)
  Brk_Liquid_Prs_mv/1 -> Analog_Signal_Process/3(Brk_Liquid_Prs_mv)
  Acc_Lft_Disp_mv/1 -> Analog_Signal_Process/1(Acc_Lft_Disp_mv)
  Acc_Right_Disp_mv/1 -> Analog_Signal_Process/2(Acc_Right_Disp_mv)
  Analog_Signal_Process/2(Acc_Right_Disp_Val) -> Acc_Right_Disp_Val/1
  Analog_Signal_Process/1(Acc_Lft_Disp_Val) -> Acc_Lft_Disp_Val/1
  Analog_Signal_Process/6(ACC) -> ACC/1

== system FSAC2021_V1/VCU_CAN_Read/PCANA(RES、AMI、MOTEC、BRAKE、STEER_SENSOR、IPC) ==
  function : TriggerPort  TriggerType=function-call
  BCU_MTR_STATUS : ec55xxlib/RapidECU_U2/07CANCommucation/CANReceive  canmodule=A  canbuffer=21  canmessageid=257  canmessagetype=Standard(11-bit ID)  datalength=8  sampletime=-1
  BCU_MTR_STATUS1 : Subsystem
  Data Type Conversion{1..21} (21 alike) : DataTypeConversion
  IPC_CMD1 : Subsystem
  MOTEC_MOTION1 : ec55xxlib/RapidECU_U2/07CANCommucation/CANReceive  canmodule=A  canbuffer=41  canmessageid=256  canmessagetype=Standard(11-bit ID)  datalength=3  sampletime=-1
  MOTEC_MOTION2 : ec55xxlib/RapidECU_U2/07CANCommucation/CANReceive  canmodule=A  canbuffer=35  canmessageid=279  canmessagetype=Standard(11-bit ID)  datalength=1  sampletime=-1
  MeaModule2 : ec55xxlib/RapidECU_U2/11Calibration/MeaModule  signal=brake_node
  MeaModule3 : ec55xxlib/RapidECU_U2/11Calibration/MeaModule  signal=strsr_node
  MeaModule4 : ec55xxlib/RapidECU_U2/11Calibration/MeaModule  signal=RES_Value
  MeaModule5 : ec55xxlib/RapidECU_U2/11Calibration/MeaModule  signal=RES__ok
  MeaModule6 : ec55xxlib/RapidECU_U2/11Calibration/MeaModule  signal=Steer_sensor_angle
  Res_Message1 : Subsystem
  STEER_SENSOR_INFO1 : Subsystem
  Steer_Sensor : ec55xxlib/RapidECU_U2/07CANCommucation/CANReceive  canmodule=A  canbuffer=38  canmessageid=485  canmessagetype=Standard(11-bit ID)  datalength=8  sampletime=-1
  Subsystem : Subsystem
  Terminator{1,3,11,13..20} (11 alike) : Terminator
  StrSr_Node : Outport
  StrSr_Snr_Ang : Outport  Port=2
  Brake_mtr_goalpos_Out : Outport  Port=3
  Brake_speed_enqual_Out : Outport  Port=4
  Brake_pos_enqual_Out : Outport  Port=5
  Brake_sensor6_sts_Out : Outport  Port=6
  Brake_sensor5_sts_Out : Outport  Port=7
  Brake_sensor4_sts_Out : Outport  Port=8
  Brake_sensor3_sts_Out : Outport  Port=9
  Brake_sensor2_sts_Out : Outport  Port=10
  Brake_sensor1_sts_Out : Outport  Port=11
  Brake_reg_rw_fault_flag_Out : Outport  Port=12
  Brake_overheat_prtct_sts_Out : Outport  Port=13
  Brake_overcurrt_prtct_sts_Out : Outport  Port=14
  Brake_offline_run_flag_O : Outport  Port=15
  Brake_mtr_stop_flag_Out : Outport  Port=16
  Brake_mtr_origin_flag_Out : Outport  Port=17
  Brake_mtr_enable_flag_Out : Outport  Port=18
  Brake_lowvolt_prtct_sts_Out : Outport  Port=19
  Brake_hd_fault_sts_Out : Outport  Port=20
  Brake_go_origin_over_flag_Out : Outport  Port=21
  Brake_encoder_fault_sts_Out : Outport  Port=22
  Brake_cmd_fault_flag_Out : Outport  Port=23
  Brk_Node : Outport  Port=24
  IPC_Steer : Outport  Port=25
  IPC_Brk : Outport  Port=26
  IPC_Acc : Outport  Port=27
  RES_Signal : Outport  Port=28
  wires:
  Steer_Sensor/1 -> STEER_SENSOR_INFO1/Trigger
  Steer_Sensor/4 -> STEER_SENSOR_INFO1/1(input)
  Steer_Sensor/2 -> MeaModule3/1
  STEER_SENSOR_INFO1/1(Str_Sensor_Curr_Angle_Out) -> MeaModule6/1
  Steer_Sensor/3 -> Terminator11/1
  Steer_Sensor/5 -> Terminator15/1
  MeaModule3/1 -> StrSr_Node/1
  MeaModule6/1 -> StrSr_Snr_Ang/1
  BCU_MTR_STATUS1/13(Brake_offline_run_flag_Out) -> Data Type Conversion13/1
  BCU_MTR_STATUS1/2(Brake_speed_enqual_Out) -> Data Type Conversion2/1
  BCU_MTR_STATUS/5 -> Terminator20/1
  BCU_MTR_STATUS1/16(Brake_mtr_enable_flag_Out) -> Data Type Conversion16/1
  BCU_MTR_STATUS/3 -> Terminator19/1
  BCU_MTR_STATUS/2 -> MeaModule2/1
  BCU_MTR_STATUS1/5(Brake_sensor5_sts_Out) -> Data Type Conversion5/1
  BCU_MTR_STATUS1/14(Brake_mtr_stop_flag_Out) -> Data Type Conversion14/1
  BCU_MTR_STATUS1/17(Brake_lowvolt_prtct_sts_Out) -> Data Type Conversion17/1
  BCU_MTR_STATUS/4 -> BCU_MTR_STATUS1/1(input)
  BCU_MTR_STATUS1/1(Brake_mtr_goalpos_Out) -> Data Type Conversion1/1
  BCU_MTR_STATUS1/18(Brake_hd_fault_sts_Out) -> Data Type Conversion18/1
  BCU_MTR_STATUS1/12(Brake_overcurrt_prtct_sts_Out) -> Data Type Conversion12/1
  BCU_MTR_STATUS1/19(Brake_go_origin_over_flag_Out) -> Data Type Conversion19/1
  BCU_MTR_STATUS/1 -> BCU_MTR_STATUS1/Trigger
  BCU_MTR_STATUS1/6(Brake_sensor4_sts_Out) -> Data Type Conversion6/1
  BCU_MTR_STATUS1/4(Brake_sensor6_sts_Out) -> Data Type Conversion4/1
  BCU_MTR_STATUS1/8(Brake_sensor2_sts_Out) -> Data Type Conversion8/1
  BCU_MTR_STATUS1/3(Brake_pos_enqual_Out) -> Data Type Conversion3/1
  BCU_MTR_STATUS1/10(Brake_reg_rw_fault_flag_Out) -> Data Type Conversion10/1
  BCU_MTR_STATUS1/20(Brake_encoder_fault_sts_Out) -> Data Type Conversion20/1
  BCU_MTR_STATUS1/21(Brake_cmd_fault_flag_Out) -> Data Type Conversion21/1
  BCU_MTR_STATUS1/9(Brake_sensor1_sts_Out) -> Data Type Conversion9/1
  BCU_MTR_STATUS1/15(Brake_mtr_origin_flag_Out) -> Data Type Conversion15/1
  BCU_MTR_STATUS1/11(Brake_overheat_prtct_sts_Out) -> Data Type Conversion11/1
  BCU_MTR_STATUS1/7(Brake_sensor3_sts_Out) -> Data Type Conversion7/1
  Data Type Conversion17/1 -> Brake_lowvolt_prtct_sts_Out/1
  Data Type Conversion1/1 -> Brake_mtr_goalpos_Out/1
  Data Type Conversion11/1 -> Brake_overheat_prtct_sts_Out/1
  Data Type Conversion13/1 -> Brake_offline_run_flag_O/1
  Data Type Conversion12/1 -> Brake_overcurrt_prtct_sts_Out/1
  Data Type Conversion10/1 -> Brake_reg_rw_fault_flag_Out/1
  Data Type Conversion16/1 -> Brake_mtr_enable_flag_Out/1
  Data Type Conversion14/1 -> Brake_mtr_stop_flag_Out/1
  Data Type Conversion18/1 -> Brake_hd_fault_sts_Out/1
  Data Type Conversion4/1 -> Brake_sensor6_sts_Out/1
  Data Type Conversion5/1 -> Brake_sensor5_sts_Out/1
  Data Type Conversion6/1 -> Brake_sensor4_sts_Out/1
  Data Type Conversion7/1 -> Brake_sensor3_sts_Out/1
  Data Type Conversion15/1 -> Brake_mtr_origin_flag_Out/1
  Data Type Conversion2/1 -> Brake_speed_enqual_Out/1
  Data Type Conversion8/1 -> Brake_sensor2_sts_Out/1
  Data Type Conversion19/1 -> Brake_go_origin_over_flag_Out/1
  Data Type Conversion9/1 -> Brake_sensor1_sts_Out/1
  Data Type Conversion21/1 -> Brake_cmd_fault_flag_Out/1
  Data Type Conversion3/1 -> Brake_pos_enqual_Out/1
  Data Type Conversion20/1 -> Brake_encoder_fault_sts_Out/1
  MeaModule2/1 -> Brk_Node/1
  MOTEC_MOTION1/4 -> IPC_CMD1/1(input)
  MOTEC_MOTION1/1 -> IPC_CMD1/Trigger
  MOTEC_MOTION1/3 -> Terminator3/1
  MOTEC_MOTION1/5 -> Terminator13/1
  Subsystem/3(Out3) -> IPC_Acc/1
  Subsystem/2(Out2) -> IPC_Brk/1
  IPC_CMD1/1(IPC_Steer_Out) -> Subsystem/1(In1)
  IPC_CMD1/2(IPC_Brk_Out) -> Subsystem/2(In2)
  IPC_CMD1/3(IPC_Acc_Out) -> Subsystem/3(In3)
  MOTEC_MOTION1/2 -> Subsystem/Enable
  Subsystem/1(Out1) -> IPC_Steer/1
  MOTEC_MOTION2/1 -> Res_Message1/Trigger
  MOTEC_MOTION2/2 -> MeaModule5/1
  MOTEC_MOTION2/3 -> Terminator14/1
  MOTEC_MOTION2/4 -> Res_Message1/1(input)
  MOTEC_MOTION2/5 -> Terminator16/1
  Res_Message1/1(Safety_Relay_Out) -> Terminator17/1
  Res_Message1/3(Res_check_Out) -> Terminator18/1
  Res_Message1/2(Res_Run_Status_Out) -> MeaModule4/1
  MeaModule4/1 -> RES_Signal/1
  MeaModule5/1 -> Terminator1/1

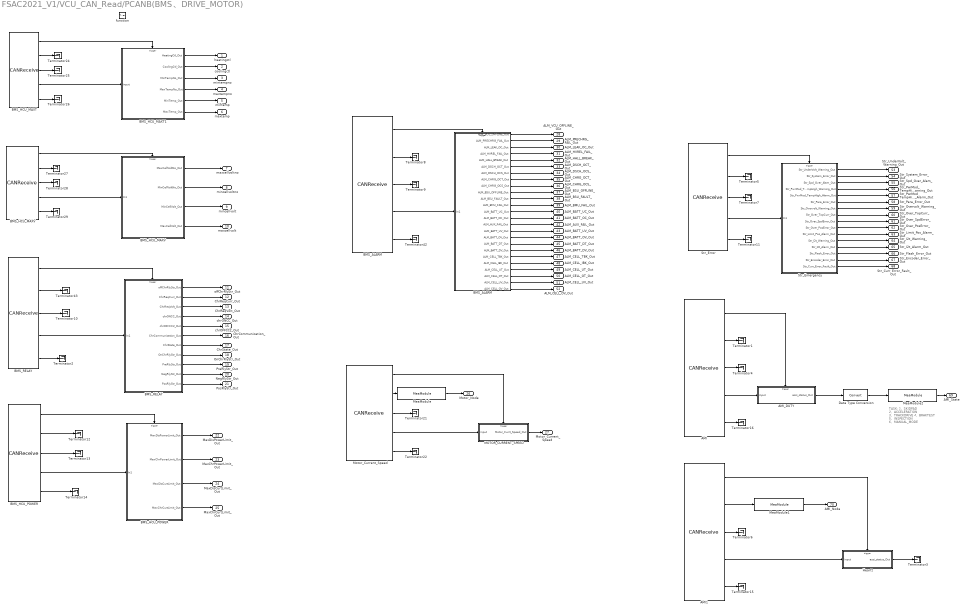
== system FSAC2021_V1/VCU_CAN_Read/PCANB(BMS、DRIVE_MOTOR) ==
  note: TASK:
      | 1、SKIDPAD
      | 2、ACCELERATION
      | 3、TRACKDRIVE
      | 4、BRAKTEST
      | 5、INSPECTION
      | 6、MANUAL_MODE
  function : TriggerPort  TriggerType=function-call
  AMI : ec55xxlib/RapidECU_U2/07CANCommucation/CANReceive  canmodule=A  canbuffer=16  canmessageid=1169  canmessagetype=Standard(11-bit ID)  datalength=1  sampletime=-1
  AMI1 : ec55xxlib/RapidECU_U2/07CANCommucation/CANReceive  canmodule=A  canbuffer=26  canmessageid=1168  canmessagetype=Standard(11-bit ID)  datalength=1  sampletime=-1
  AMI_DUTY : Subsystem
  BMS_ALARM : ec55xxlib/RapidECU_U2/07CANCommucation/CANReceive  canmodule=B  canbuffer=50  canmessageid=2556772595  canmessagetype=Extended(29-bit ID)  datalength=8  sampletime=-1
  "BMS_ALARM " : Subsystem
  BMS_HCU_MAXT : ec55xxlib/RapidECU_U2/07CANCommucation/CANReceive  canmodule=B  canbuffer=18  canmessageid=2556575987  canmessagetype=Extended(29-bit ID)  datalength=8  sampletime=-1
  BMS_HCU_MAXT1 : Subsystem
  BMS_HCU_MAXV : ec55xxlib/RapidECU_U2/07CANCommucation/CANReceive  canmodule=B  canbuffer=16  canmessageid=2556510451  canmessagetype=Extended(29-bit ID)  datalength=8  sampletime=-1
  "BMS_HCU_MAXV " : Subsystem
  BMS_HCU_POWER : ec55xxlib/RapidECU_U2/07CANCommucation/CANReceive  canmodule=B  canbuffer=52  canmessageid=2556707059  canmessagetype=Extended(29-bit ID)  datalength=8  sampletime=-1
  "BMS_HCU_POWER " : Subsystem
  BMS_RELAY : ec55xxlib/RapidECU_U2/07CANCommucation/CANReceive  canmodule=B  canbuffer=51  canmessageid=2556641523  canmessagetype=Extended(29-bit ID)  datalength=8  sampletime=-1
  "BMS_RELAY " : Subsystem
  Data Type Conversion : DataTypeConversion
  Heartt : Subsystem
  MOTOR_CURRENT_SPEED : Subsystem
  MeaModule : ec55xxlib/RapidECU_U2/11Calibration/MeaModule  signal=motor_node
  MeaModule1 : ec55xxlib/RapidECU_U2/11Calibration/MeaModule  signal=AMI_HEART
  MeaModule2 : ec55xxlib/RapidECU_U2/11Calibration/MeaModule  signal=AMI
  "Motor_Current_Speed " : ec55xxlib/RapidECU_U2/07CANCommucation/CANReceive  canmodule=B  canbuffer=21  canmessageid=2147553443  canmessagetype=Extended(29-bit ID)  datalength=2  sampletime=-1
  "Str_Emergency " : Subsystem
  Str_Error : ec55xxlib/RapidECU_U2/07CANCommucation/CANReceive  canmodule=A  canbuffer=4  canmessageid=129  canmessagetype=Standard(11-bit ID)  datalength=8  sampletime=-1
  Terminator{1..16,21..22,24..29,42..43} (26 alike) : Terminator
  heatingctl : Outport
  coolingctl : Outport  Port=2
  mintempno : Outport  Port=3
  maxtempno : Outport  Port=4
  mintemp : Outport  Port=5
  maxtemp : Outport  Port=6
  maxcellvoltno : Outport  Port=7
  mincellvoltno : Outport  Port=8
  mincellvolt : Outport  Port=9
  maxcellvolt : Outport  Port=10
  offChrRlyStr_Out : Outport  Port=11
  ChrReqCurr_Out : Outport  Port=12
  ChrReqVolt_Out : Outport  Port=13
  chrONCC_Out : Outport  Port=14
  chrOFFCC2_Out : Outport  Port=15
  ChrCommunication_Out : Outport  Port=16
  ChrState_Out : Outport  Port=17
  OnChrRlyStr_Out : Outport  Port=18
  PreRlyStr_Out : Outport  Port=19
  NegRlyStr_Out : Outport  Port=20
  PosRlyStr_Out : Outport  Port=21
  MaxDisPowerLimit_Out : Outport  Port=22
  MaxChrPowerLimit_Out : Outport  Port=23
  MaxDisCurtLimit_Out : Outport  Port=24
  MaxChrCurtLimit_Out : Outport  Port=25
  Motor_Node : Outport  Port=26
  Motor_Current_Speed : Outport  Port=27
  ALM_VCU_OFFLINE_Out : Outport  Port=28
  ALM_PRECHRG_FAIL_Out : Outport  Port=29
  ALM_LEAK_OC_Out : Outport  Port=30
  ALM_HVREL_FAIL_Out : Outport  Port=31
  ALM_HALL_BREAK_Out : Outport  Port=32
  ALM_DSCH_OCT_Out : Outport  Port=33
  ALM_DSCH_OCS_Out : Outport  Port=34
  ALM_CHRG_OCT_Out : Outport  Port=35
  ALM_CHRG_OCS_Out : Outport  Port=36
  ALM_BSU_OFFLINE_Out : Outport  Port=37
  ALM_BSU_FAULT_Out : Outport  Port=38
  ALM_BMU_FAIL_Out : Outport  Port=39
  ALM_BATT_UC_Out : Outport  Port=40
  ALM_BATT_OC_Out : Outport  Port=41
  ALM_AUX_FAIL_Out : Outport  Port=42
  ALM_BATT_UV_Out : Outport  Port=43
  ALM_BATT_OV_Out : Outport  Port=44
  ALM_BATT_DT_Out : Outport  Port=45
  ALM_BATT_DV_Out : Outport  Port=46
  ALM_CELL_TBK_Out : Outport  Port=47
  ALM_CELL_IBK_Out : Outport  Port=48
  ALM_CELL_UT_Out : Outport  Port=49
  ALM_CELL_OT_Out : Outport  Port=50
  ALM_CELL_UV_Out : Outport  Port=51
  ALM_CELL_OV_Out : Outport  Port=52
  Str_UnderVolt_Warning_Out : Outport  Port=53
  Str_System_Error_Out : Outport  Port=54
  Str_Spd_Over_Alam_Out : Outport  Port=55
  Str_PwrMod_TempHigh_Warning_Out : Outport  Port=56
  Str_PwrMod_TempHigh_Alarm_Out : Outport  Port=57
  Str_Para_Error_Out : Outport  Port=58
  Str_Overvolt_Warning_Out : Outport  Port=59
  Str_Over_TopCurr_Out : Outport  Port=60
  Str_Over_SpdError_Out : Outport  Port=61
  Str_Over_PosError_Out : Outport  Port=62
  Str_Limit_Pos_Alarm_Out : Outport  Port=63
  Str_I2t_Warning_Out : Outport  Port=64
  Str_I2t_Alarm_Out : Outport  Port=65
  Str_Flash_Error_Out : Outport  Port=66
  Str_Encoder_Error_Out : Outport  Port=67
  Str_Curr_Error_Fault_Out : Outport  Port=68
  AMI_State : Outport  Port=69
  AMI_Node : Outport  Port=70
  wires:
  BMS_ALARM/5 -> Terminator42/1
  BMS_ALARM/1 -> "BMS_ALARM "/Trigger
  BMS_ALARM/3 -> Terminator9/1
  BMS_ALARM/2 -> Terminator8/1
  BMS_ALARM/4 -> "BMS_ALARM "/1(In1)
  BMS_RELAY/1 -> "BMS_RELAY "/Trigger
  BMS_RELAY/3 -> Terminator10/1
  BMS_RELAY/4 -> "BMS_RELAY "/1(In1)
  BMS_RELAY/5 -> Terminator2/1
  BMS_RELAY/2 -> Terminator43/1
  BMS_HCU_POWER/5 -> Terminator14/1
  BMS_HCU_POWER/2 -> Terminator12/1
  BMS_HCU_POWER/4 -> "BMS_HCU_POWER "/1(In1)
  BMS_HCU_POWER/3 -> Terminator13/1
  BMS_HCU_MAXT/3 -> Terminator25/1
  BMS_HCU_MAXT/2 -> Terminator24/1
  BMS_HCU_MAXT/5 -> Terminator26/1
  BMS_HCU_MAXT/1 -> BMS_HCU_MAXT1/Trigger
  BMS_HCU_MAXT/4 -> BMS_HCU_MAXT1/1(input)
  BMS_HCU_MAXV/4 -> "BMS_HCU_MAXV "/1(In1)
  BMS_HCU_MAXV/3 -> Terminator28/1
  BMS_HCU_MAXV/1 -> "BMS_HCU_MAXV "/Trigger
  BMS_HCU_MAXV/5 -> Terminator29/1
  BMS_HCU_MAXV/2 -> Terminator27/1
  BMS_HCU_POWER/1 -> "BMS_HCU_POWER "/Trigger
  "Motor_Current_Speed "/4 -> MOTOR_CURRENT_SPEED/1(input)
  "Motor_Current_Speed "/1 -> MOTOR_CURRENT_SPEED/Trigger
  "Motor_Current_Speed "/2 -> MeaModule/1
  "Motor_Current_Speed "/3 -> Terminator21/1
  "Motor_Current_Speed "/5 -> Terminator22/1
  BMS_HCU_MAXT1/1(HeatingCtl_Out) -> heatingctl/1
  BMS_HCU_MAXT1/2(CoolingCtl_Out) -> coolingctl/1
  BMS_HCU_MAXT1/3(MinTempNo_Out) -> mintempno/1
  BMS_HCU_MAXT1/4(MaxTempNo_Out) -> maxtempno/1
  BMS_HCU_MAXT1/5(MinTemp_Out) -> mintemp/1
  BMS_HCU_MAXT1/6(MaxTemp_Out) -> maxtemp/1
  "BMS_HCU_MAXV "/1(MaxCellVoltNo_Out) -> maxcellvoltno/1
  "BMS_HCU_MAXV "/3(MinCellVolt_Out) -> mincellvolt/1
  "BMS_HCU_MAXV "/4(MaxCellVolt_Out) -> maxcellvolt/1
  "BMS_HCU_MAXV "/2(MinCellVoltNo_Out) -> mincellvoltno/1
  "BMS_RELAY "/1(offChrRlyStr_Out) -> offChrRlyStr_Out/1
  "BMS_RELAY "/2(ChrReqCurr_Out) -> ChrReqCurr_Out/1
  "BMS_RELAY "/3(ChrReqVolt_Out) -> ChrReqVolt_Out/1
  "BMS_RELAY "/4(chrONCC_Out) -> chrONCC_Out/1
  "BMS_RELAY "/5(chrOFFCC2_Out) -> chrOFFCC2_Out/1
  "BMS_RELAY "/10(NegRlyStr_Out) -> NegRlyStr_Out/1
  "BMS_RELAY "/9(PreRlyStr_Out) -> PreRlyStr_Out/1
  "BMS_RELAY "/11(PosRlyStr_Out) -> PosRlyStr_Out/1
  "BMS_RELAY "/6(ChrCommunication_Out) -> ChrCommunication_Out/1
  "BMS_RELAY "/8(OnChrRlyStr_Out) -> OnChrRlyStr_Out/1
  "BMS_RELAY "/7(ChrState_Out) -> ChrState_Out/1
  "BMS_HCU_POWER "/3(MaxDisCurtLimit_Out) -> MaxDisCurtLimit_Out/1
  "BMS_HCU_POWER "/4(MaxChrCurtLimit_Out) -> MaxChrCurtLimit_Out/1
  "BMS_HCU_POWER "/1(MaxDisPowerLimit_Out) -> MaxDisPowerLimit_Out/1
  "BMS_HCU_POWER "/2(MaxChrPowerLimit_Out) -> MaxChrPowerLimit_Out/1
  MeaModule/1 -> Motor_Node/1
  MOTOR_CURRENT_SPEED/1(Motor_Currt_Speed_Out) -> Motor_Current_Speed/1
  "BMS_ALARM "/20(ALM_CELL_TBK_Out) -> ALM_CELL_TBK_Out/1
  "BMS_ALARM "/21(ALM_CELL_IBK_Out) -> ALM_CELL_IBK_Out/1
  "BMS_ALARM "/13(ALM_BATT_UC_Out) -> ALM_BATT_UC_Out/1
  "BMS_ALARM "/1(ALM_VCU_OFFLINE_Out) -> ALM_VCU_OFFLINE_Out/1
  "BMS_ALARM "/9(ALM_CHRG_OCS_Out) -> ALM_CHRG_OCS_Out/1
  "BMS_ALARM "/22(ALM_CELL_UT_Out) -> ALM_CELL_UT_Out/1
  "BMS_ALARM "/14(ALM_BATT_OC_Out) -> ALM_BATT_OC_Out/1
  "BMS_ALARM "/15(ALM_AUX_FAIL_Out) -> ALM_AUX_FAIL_Out/1
  "BMS_ALARM "/2(ALM_PRECHRG_FAIL_Out) -> ALM_PRECHRG_FAIL_Out/1
  "BMS_ALARM "/6(ALM_DSCH_OCT_Out) -> ALM_DSCH_OCT_Out/1
  "BMS_ALARM "/7(ALM_DSCH_OCS_Out) -> ALM_DSCH_OCS_Out/1
  "BMS_ALARM "/5(ALM_HALL_BREAK_Out) -> ALM_HALL_BREAK_Out/1
  "BMS_ALARM "/8(ALM_CHRG_OCT_Out) -> ALM_CHRG_OCT_Out/1
  "BMS_ALARM "/12(ALM_BMU_FAIL_Out) -> ALM_BMU_FAIL_Out/1
  "BMS_ALARM "/16(ALM_BATT_UV_Out) -> ALM_BATT_UV_Out/1
  "BMS_ALARM "/17(ALM_BATT_OV_Out) -> ALM_BATT_OV_Out/1
  "BMS_ALARM "/4(ALM_HVREL_FAIL_Out) -> ALM_HVREL_FAIL_Out/1
  "BMS_ALARM "/18(ALM_BATT_DT_Out) -> ALM_BATT_DT_Out/1
  "BMS_ALARM "/11(ALM_BSU_FAULT_Out) -> ALM_BSU_FAULT_Out/1
  "BMS_ALARM "/10(ALM_BSU_OFFLINE_Out) -> ALM_BSU_OFFLINE_Out/1
  "BMS_ALARM "/19(ALM_BATT_DV_Out) -> ALM_BATT_DV_Out/1
  "BMS_ALARM "/3(ALM_LEAK_OC_Out) -> ALM_LEAK_OC_Out/1
  "BMS_ALARM "/24(ALM_CELL_UV_Out) -> ALM_CELL_UV_Out/1
  "BMS_ALARM "/25(ALM_CELL_OV_Out) -> ALM_CELL_OV_Out/1
  "BMS_ALARM "/23(ALM_CELL_OT_Out) -> ALM_CELL_OT_Out/1
  AMI/2 -> Terminator1/1
  AMI/5 -> Terminator16/1
  AMI/1 -> AMI_DUTY/Trigger
  AMI_DUTY/1(assi_status_Out) -> Data Type Conversion/1
  Data Type Conversion/1 -> MeaModule2/1
  AMI/4 -> AMI_DUTY/1(input)
  AMI/3 -> Terminator4/1
  AMI1/4 -> Heartt/1(input)
  AMI1/3 -> Terminator6/1
  AMI1/5 -> Terminator15/1
  AMI1/1 -> Heartt/Trigger
  AMI1/2 -> MeaModule1/1
  Heartt/1(assi_status_Out) -> Terminator3/1
  "Str_Emergency "/3(Str_Spd_Over_Alam_Out) -> Str_Spd_Over_Alam_Out/1
  "Str_Emergency "/15(Str_Encoder_Error_Out) -> Str_Encoder_Error_Out/1
  "Str_Emergency "/2(Str_System_Error_Out) -> Str_System_Error_Out/1
  "Str_Emergency "/13(Str_I2t_Alarm_Out) -> Str_I2t_Alarm_Out/1
  "Str_Emergency "/6(Str_Para_Error_Out) -> Str_Para_Error_Out/1
  "Str_Emergency "/5(Str_PwrMod_TempHigh_Alarm_Out) -> Str_PwrMod_TempHigh_Alarm_Out/1
  "Str_Emergency "/12(Str_I2t_Warning_Out) -> Str_I2t_Warning_Out/1
  Str_Error/5 -> Terminator11/1
  "Str_Emergency "/10(Str_Over_PosError_Out) -> Str_Over_PosError_Out/1
  Str_Error/4 -> "Str_Emergency "/1(In1)
  Str_Error/2 -> Terminator5/1
  "Str_Emergency "/7(Str_Overvolt_Warning_Out) -> Str_Overvolt_Warning_Out/1
  "Str_Emergency "/1(Str_UnderVolt_Warning_Out) -> Str_UnderVolt_Warning_Out/1
  "Str_Emergency "/11(Str_Limit_Pos_Alarm_Out) -> Str_Limit_Pos_Alarm_Out/1
  "Str_Emergency "/9(Str_Over_SpdError_Out) -> Str_Over_SpdError_Out/1
  Str_Error/3 -> Terminator7/1
  "Str_Emergency "/4(Str_PwrMod_TempHigh_Warning_Out) -> Str_PwrMod_TempHigh_Warning_Out/1
  "Str_Emergency "/16(Str_Curr_Error_Fault_Out) -> Str_Curr_Error_Fault_Out/1
  "Str_Emergency "/8(Str_Over_TopCurr_Out) -> Str_Over_TopCurr_Out/1
  "Str_Emergency "/14(Str_Flash_Error_Out) -> Str_Flash_Error_Out/1
  Str_Error/1 -> "Str_Emergency "/Trigger
  MeaModule2/1 -> AMI_State/1
  MeaModule1/1 -> AMI_Node/1

== system FSAC2021_V1/VCU_CAN_Read/Subsystem ==
  function : TriggerPort  TriggerType=function-call
  BMS_HCU_INFO : ec55xxlib/RapidECU_U2/07CANCommucation/CANReceive  canmodule=B  canbuffer=54  canmessageid=2556444915  canmessagetype=Extended(29-bit ID)  datalength=8  sampletime=-1
  "BMS_HCU_INFO " : Subsystem
  MeaModule1 : ec55xxlib/RapidECU_U2/11Calibration/MeaModule  signal=bms_node
  Terminator16 : Terminator
  Terminator17 : Terminator
  BATLIFE : Outport
  BATALM : Outport  Port=2
  BATSTATE : Outport  Port=3
  BATSOH : Outport  Port=4
  BATSOC : Outport  Port=5
  BATCURRENT : Outport  Port=6
  BATVOLTAGLE : Outport  Port=7
  BMS_NODE : Outport  Port=8
  wires:
  "BMS_HCU_INFO "/7(BatVoltage_Out) -> BATVOLTAGLE/1
  "BMS_HCU_INFO "/6(BatCurrent_Out) -> BATCURRENT/1
  BMS_HCU_INFO/1 -> "BMS_HCU_INFO "/Trigger
  "BMS_HCU_INFO "/1(BatLife_Out) -> BATLIFE/1
  BMS_HCU_INFO/3 -> Terminator16/1
  "BMS_HCU_INFO "/5(BatSoc_Out) -> BATSOC/1
  "BMS_HCU_INFO "/2(BatAlmLv_Out) -> BATALM/1
  BMS_HCU_INFO/5 -> Terminator17/1
  "BMS_HCU_INFO "/3(BatState_Out) -> BATSTATE/1
  BMS_HCU_INFO/4 -> "BMS_HCU_INFO "/1(In1)
  BMS_HCU_INFO/2 -> MeaModule1/1
  "BMS_HCU_INFO "/4(BatSoh_Out) -> BATSOH/1
  MeaModule1/1 -> BMS_NODE/1
